simulink library "SUB_PLANT_Engine"  (R2018a)
settings: Solver=VariableStepAuto  StartTime=0.0  StopTime=10.0  RelTol=1e-3
libraries: PTC_MBDS_LIB x19, simulink x9
settings Model: Creator=Sundeep.Tuteja  LastModifiedBy=John.Lahti

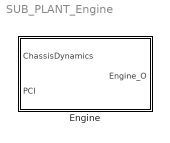
== system SUB_PLANT_Engine ==
  Engine : Subsystem

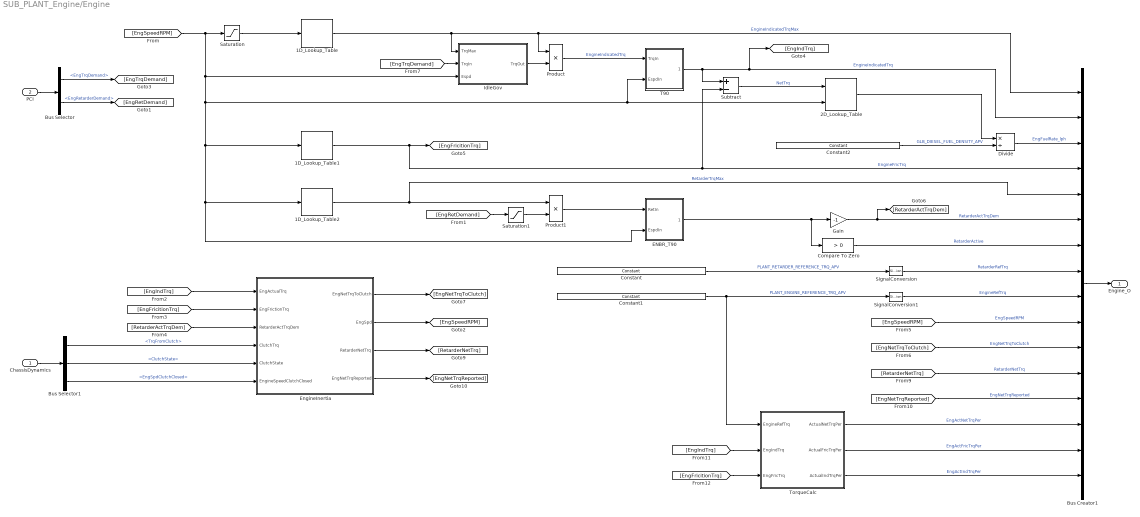
== system SUB_PLANT_Engine/Engine ==
  ChassisDynamics : Inport
  PCI : Inport  Port=2
  1D_Lookup_Table : PTC_MBDS_LIB/Extras/Lookup Tables/1D_Lookup_Table  ParameterObjectName=PLANT_ENGINE_INDICATED_TORQUE_DATA_MPV  InterpolationMethod=Linear  PTC_MBDS_BlockVersion=5.41  PTC_BlockType=PTC_MBDS_1D_Lookup_Table
      settings: SourceProductName=PACCAR Technical Center MBDS Library
      settings: AttributesFormatString=|
      | X Axis: PLANT_ENGINE_INDICATED_TORQUE_STEP_MPV (rpm)
      | Y Axis: PLANT_ENGINE_INDICATED_TORQUE_DATA_MPV (N*m)
      | Interpolation Method: Linear
  1D_Lookup_Table1 : PTC_MBDS_LIB/Extras/Lookup Tables/1D_Lookup_Table  ParameterObjectName=PLANT_ENGINE_FRICTION_TORQUE_DATA_MPV  InterpolationMethod=Linear  PTC_MBDS_BlockVersion=5.41  PTC_BlockType=PTC_MBDS_1D_Lookup_Table
      settings: SourceProductName=PACCAR Technical Center MBDS Library
      settings: AttributesFormatString=|
      | X Axis: PLANT_ENGINE_FRICTION_TORQUE_STEP_MPV (rpm)
      | Y Axis: PLANT_ENGINE_FRICTION_TORQUE_DATA_MPV (N*m)
      | Interpolation Method: Linear
  1D_Lookup_Table2 : PTC_MBDS_LIB/Extras/Lookup Tables/1D_Lookup_Table  ParameterObjectName=PLANT_RETARDER_TORQUE_DATA_MPV  InterpolationMethod=Linear  PTC_MBDS_BlockVersion=5.41  PTC_BlockType=PTC_MBDS_1D_Lookup_Table
      settings: SourceProductName=PACCAR Technical Center MBDS Library
      settings: AttributesFormatString=|
      | X Axis: PLANT_RETARDER_TORQUE_STEP_MPV (rpm)
      | Y Axis: PLANT_RETARDER_TORQUE_DATA_MPV (N*m)
      | Interpolation Method: Linear
  2D_Lookup_Table : PTC_MBDS_LIB/Extras/Lookup Tables/2D_Lookup_Table  ParameterObjectName=PLANT_ENGINE_FUEL_MAP_DATA_MPV  InterpolationMethod=Linear  PTC_MBDS_BlockVersion=5.41  PTC_BlockType=PTC_MBDS_2D_Lookup_Table
      settings: SourceProductName=PACCAR Technical Center MBDS Library
      settings: AttributesFormatString=|
      | Row Axis: PLANT_ENGINE_FUEL_MAP_TRQ_STEP_MPV (N*m)
      | Column Axis: PLANT_ENGINE_FUEL_MAP_ESPD_STEP_MPV (rpm)
      | Data Axis: PLANT_ENGINE_FUEL_MAP_DATA_MPV (kg/h)
      | Interpolation Method: Linear
  Bus Creator1 : BusCreator  Inputs=16
  Bus Selector : BusSelector  OutputSignals=EngTrqDemand,EngRetarderDemand
  Bus Selector1 : BusSelector  OutputSignals=Chassis.TrqFromClutch,Chassis.ClutchState,Chassis.EngSpdClutchClosed
  Compare To Zero : simulink/Logic and Bit Operations/Compare To Zero  relop=>  OutDataTypeStr=boolean
  Constant : PTC_MBDS_LIB/Extras/Sources/Constant  Value2=PLANT_RETARDER_REFERENCE_TRQ_APV  PTC_MBDS_BlockVersion=5.41  PTC_BlockType=PTC_MBDS_Constant
      settings: SourceProductName=PACCAR Technical Center MBDS Library
      settings: AttributesFormatString=|
      | Value: 1779
      | Unit: 'N*m'
  Constant1 : PTC_MBDS_LIB/Extras/Sources/Constant  Value2=PLANT_ENGINE_REFERENCE_TRQ_APV  PTC_MBDS_BlockVersion=5.41  PTC_BlockType=PTC_MBDS_Constant
      settings: SourceProductName=PACCAR Technical Center MBDS Library
      settings: AttributesFormatString=|
      | Value: 2374
      | Unit: 'N*m'
  Constant2 : PTC_MBDS_LIB/Extras/Sources/Constant  Value2=GLB_DIESEL_FUEL_DENSITY_APV  PTC_MBDS_BlockVersion=5.41  PTC_BlockType=PTC_MBDS_Constant
      settings: SourceProductName=PACCAR Technical Center MBDS Library
      settings: AttributesFormatString=|
      | Value: 0.8477
      | Unit: 'kg/L'
  Divide : Product  Inputs=*/  OutDataTypeStr=Inherit: Inherit via back propagation  SaturateOnIntegerOverflow=on  InputSameDT=on
      settings: AttributesFormatString=Saturate: %<SaturateOnIntegerOverflow>
  ENBR_T90 : Subsystem
  EngineInertia : Subsystem
  Gain : Gain  Gain=-1
  IdleGov : Subsystem
  Product : Product
  Product1 : Product
  Saturation : Saturate  UpperLimit=5000  LowerLimit=500
  Saturation1 : Saturate  UpperLimit=1  LowerLimit=0
  SignalConversion : SignalConversion  ConversionOutput=Contiguous copy  OverrideOpt=off
  SignalConversion1 : SignalConversion  ConversionOutput=Contiguous copy  OverrideOpt=off
  Subtract : Sum  Inputs=+-
  T90 : Subsystem
  TorqueCalc : Subsystem
  Engine_O : Outport
  wires:
  EngineInertia/4(EngNetTrqReported) -> [EngNetTrqReported]
  EngineInertia/3(RetarderNetTrq) -> [RetarderNetTrq]
  EngineInertia/2(EngSpd) -> [EngSpeedRPM]
  EngineInertia/1(EngNetTrqToClutch) -> [EngNetTrqToClutch]
  TorqueCalc/3(ActualIndTrqPer) -> Bus Creator1/16  "EngActIndTrqPer"
  SignalConversion1/1 -> Bus Creator1/9  "EngineRefTrq"
  SignalConversion/1 -> Bus Creator1/8  "RetarderRefTrq"
  TorqueCalc/2(ActualFricTrqPer) -> Bus Creator1/15  "EngActFricTrqPer"
  TorqueCalc/1(ActualNetTrqPer) -> Bus Creator1/14  "EngActNetTrqPer"
  [EngFricitionTrq] -> TorqueCalc/3(EngFricTrq)
  [EngIndTrq] -> TorqueCalc/2(EngIndTrq)
  [EngNetTrqReported] -> Bus Creator1/13  "EngNetTrqReported"
  [RetarderNetTrq] -> Bus Creator1/12  "RetarderNetTrq"
  [EngNetTrqToClutch] -> Bus Creator1/11  "EngNetTrqToClutch"
  [EngSpeedRPM] -> Bus Creator1/10  "EngSpeedRPM"
  Bus Selector1/3 -> EngineInertia/6(EngineSpeedClutchClosed)  "<EngSpdClutchClosed>"
  Bus Selector1/2 -> EngineInertia/5(ClutchState)  "<ClutchState>"
  Bus Selector1/1 -> EngineInertia/4(ClutchTrq)  "<TrqFromClutch>"
  ChassisDynamics/1 -> Bus Selector1/1
  [RetarderActTrqDem] -> EngineInertia/3(RetarderActTrqDem)
  [EngFricitionTrq] -> EngineInertia/2(EngFrictionTrq)
  [EngIndTrq] -> EngineInertia/1(EngActualTrq)
  1D_Lookup_Table1/1 -> Bus Creator1/4, Subtract/2, [EngFricitionTrq]  "EngineFricTrq"
  Bus Creator1/1 -> Engine_O/1
  Saturation/1 -> 1D_Lookup_Table/1
  1D_Lookup_Table/1 -> Bus Creator1/1, Product/1, IdleGov/1(TrqMax)  "EngineIndicatedTrqMax"
  1D_Lookup_Table2/1 -> Product1/1, Bus Creator1/5  "RetarderTrqMax"
  [EngRetDemand] -> Saturation1/1
  Saturation1/1 -> Product1/2
  Compare To Zero/1 -> Bus Creator1/7  "RetarderActive"
  Gain/1 -> Bus Creator1/6, [RetarderActTrqDem]  "RetarderActTrqDem"
  2D_Lookup_Table/1 -> Divide/1
  PCI/1 -> Bus Selector/1
  Bus Selector/1 -> [EngTrqDemand]  "<EngTrqDemand>"
  Bus Selector/2 -> [EngRetDemand]  "<EngRetarderDemand>"
  Subtract/1 -> 2D_Lookup_Table/1  "NetTrq"
  T90/1(TrqOut) -> [EngIndTrq], Bus Creator1/2, Subtract/1  "EngineIndicatedTrq"
  ENBR_T90/1(RetOut) -> Gain/1, Compare To Zero/1
  [EngSpeedRPM] -> Saturation/1, IdleGov/3(Espd), 2D_Lookup_Table/2, T90/2(EspdIn), 1D_Lookup_Table1/1, 1D_Lookup_Table2/1, ENBR_T90/2(EspdIn)
  Product/1 -> T90/1(TrqIn)  "EngineIndicatedTrq"
  Product1/1 -> ENBR_T90/1(RetIn)
  Divide/1 -> Bus Creator1/3  "EngFuelRate_lph"
  [EngTrqDemand] -> IdleGov/2(TrqIn)
  IdleGov/1(TrqOut) -> Product/2
  Constant/1 -> SignalConversion/1  "PLANT_RETARDER_REFERENCE_TRQ_APV"
  Constant1/1 -> TorqueCalc/1(EngineRefTrq), SignalConversion1/1  "PLANT_ENGINE_REFERENCE_TRQ_APV"
  Constant2/1 -> Divide/2  "GLB_DIESEL_FUEL_DENSITY_APV"

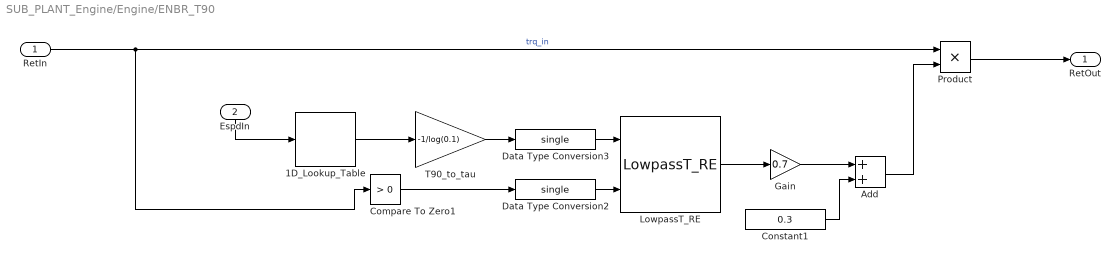
== system SUB_PLANT_Engine/Engine/ENBR_T90 ==
  RetIn : Inport
  EspdIn : Inport  Port=2
  1D_Lookup_Table : PTC_MBDS_LIB/Extras/Lookup Tables/1D_Lookup_Table  ParameterObjectName=PLANT_ENGINE_REV_T90_TIMES_MPV  InterpolationMethod=Linear  PTC_MBDS_BlockVersion=5.41  PTC_BlockType=PTC_MBDS_1D_Lookup_Table
      settings: SourceProductName=PACCAR Technical Center MBDS Library
      settings: AttributesFormatString=|
      | X Axis: PLANT_ENGINE_REV_T90_TIMES_ESPD_STEP_MPV (rpm)
      | Y Axis: PLANT_ENGINE_REV_T90_TIMES_MPV (s)
      | Interpolation Method: Linear
  Add : Sum
  Compare To Zero1 : simulink/Logic and Bit Operations/Compare To Zero  relop=>  OutDataTypeStr=boolean
  Constant1 : Constant  Value=0.3  OutDataTypeStr=single
  Data Type Conversion2 : DataTypeConversion  OutDataTypeStr=single
  Data Type Conversion3 : DataTypeConversion  OutDataTypeStr=single
  Gain : Gain  Gain=0.7
  LowpassT_RE : PTC_MBDS_LIB/MBDS Standard Library/Extended Operations/Filters/LowpassT_RE  dT_Enabled=off  dT=GLB_FIXED_STEP_SIZE_CPV  E_Enabled=off  R_Enabled=off  IV_Enabled=off  IV=0  PTC_MBDS_BlockVersion=5.41  PTC_BlockType=PTC_MBDS_LowpassT_RE
      settings: SourceProductName=PACCAR Technical Center MBDS Library
      settings: AttributesFormatString=|
      | IV = %<IV>
      | dT = %<dT>
  Product : Product
  T90_to_tau : Gain  Gain=-1/log(0.1)
  RetOut : Outport
  wires:
  Data Type Conversion2/1 -> LowpassT_RE/2
  Data Type Conversion3/1 -> LowpassT_RE/1
  1D_Lookup_Table/1 -> T90_to_tau/1
  EspdIn/1 -> 1D_Lookup_Table/1
  T90_to_tau/1 -> Data Type Conversion3/1
  Product/1 -> RetOut/1
  RetIn/1 -> Product/1, Compare To Zero1/1  "trq_in"
  Compare To Zero1/1 -> Data Type Conversion2/1
  Gain/1 -> Add/1
  Constant1/1 -> Add/2
  Add/1 -> Product/2
  LowpassT_RE/1 -> Gain/1

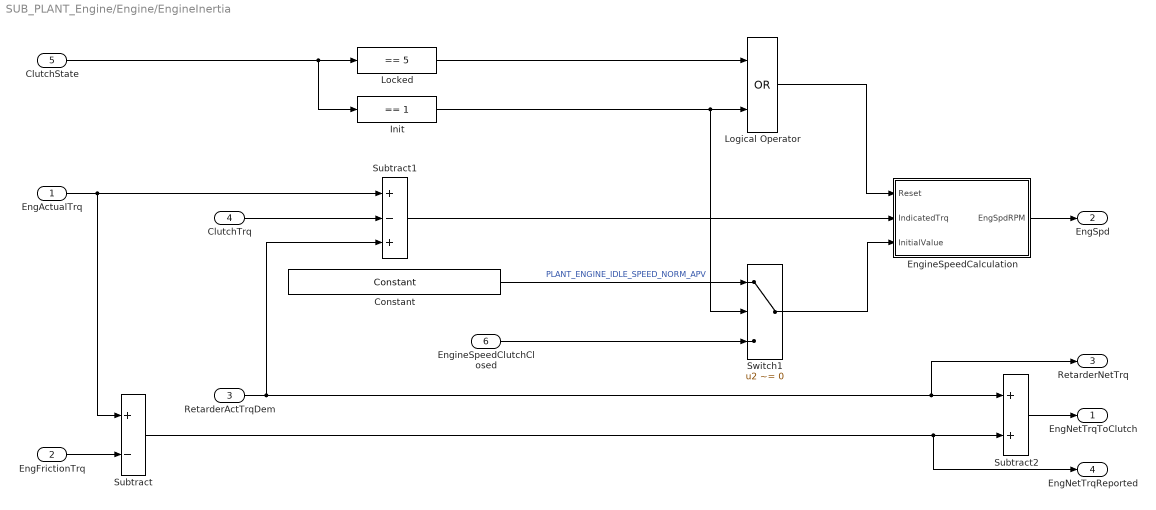
== system SUB_PLANT_Engine/Engine/EngineInertia ==
  EngActualTrq : Inport
  EngFrictionTrq : Inport  Port=2
  RetarderActTrqDem : Inport  Port=3
  ClutchTrq : Inport  Port=4
  ClutchState : Inport  Port=5
  EngineSpeedClutchClosed : Inport  Port=6
  Constant : PTC_MBDS_LIB/Extras/Sources/Constant  Value2=PLANT_ENGINE_IDLE_SPEED_NORM_APV  PTC_MBDS_BlockVersion=5.41  PTC_BlockType=PTC_MBDS_Constant
      settings: SourceProductName=PACCAR Technical Center MBDS Library
      settings: AttributesFormatString=|
      | Value: 650
      | Unit: 'rpm'
  EngineSpeedCalculation : Subsystem
  Init : simulink/Logic and Bit Operations/Compare To Constant  relop===  const=1  OutDataTypeStr=boolean
  Locked : simulink/Logic and Bit Operations/Compare To Constant  relop===  const=5  OutDataTypeStr=boolean
  Logical Operator : Logic  Operator=OR  AllPortsSameDT=off  OutDataTypeStr=boolean
  Subtract : Sum  Inputs=+-
  Subtract1 : Sum  Inputs=+-+
  Subtract2 : Sum
  Switch1 : Switch  Criteria=u2 ~= 0
  EngNetTrqToClutch : Outport
  EngSpd : Outport  Port=2
  RetarderNetTrq : Outport  Port=3
  EngNetTrqReported : Outport  Port=4
  wires:
  Constant/1 -> Switch1/1  "PLANT_ENGINE_IDLE_SPEED_NORM_APV"
  Subtract1/1 -> EngineSpeedCalculation/2(IndicatedTrq)
  RetarderActTrqDem/1 -> Subtract2/1, RetarderNetTrq/1, Subtract1/3
  Subtract2/1 -> EngNetTrqToClutch/1
  EngineSpeedCalculation/1(EngSpdRPM) -> EngSpd/1
  Logical Operator/1 -> EngineSpeedCalculation/1(Reset)
  Locked/1 -> Logical Operator/1
  ClutchState/1 -> Init/1, Locked/1
  ClutchTrq/1 -> Subtract1/2
  EngFrictionTrq/1 -> Subtract/2
  EngActualTrq/1 -> Subtract1/1, Subtract/1
  Subtract/1 -> Subtract2/2, EngNetTrqReported/1
  Init/1 -> Switch1/2, Logical Operator/2
  EngineSpeedClutchClosed/1 -> Switch1/3
  Switch1/1 -> EngineSpeedCalculation/3(InitialValue)

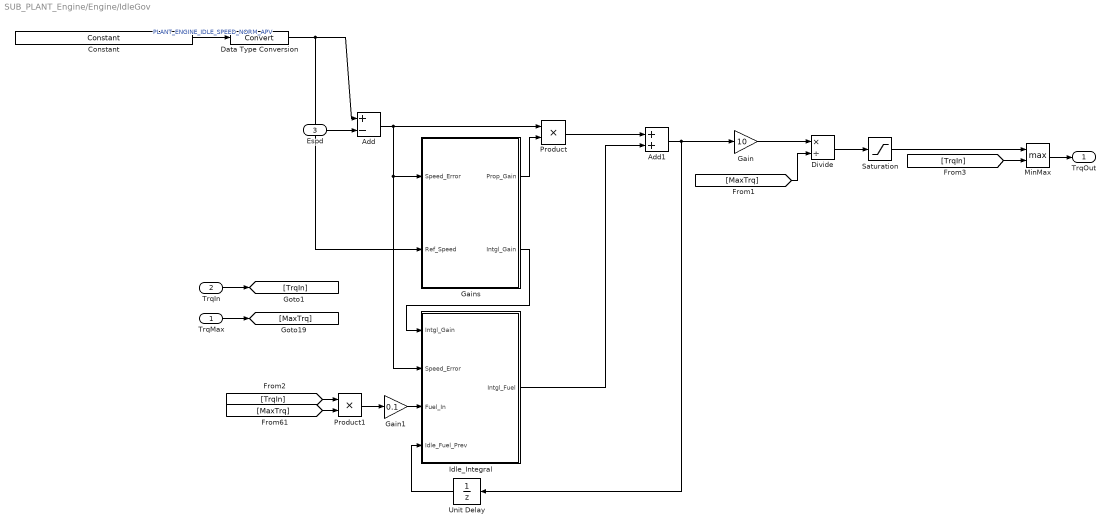
== system SUB_PLANT_Engine/Engine/IdleGov ==
  TrqMax : Inport
  TrqIn : Inport  Port=2
  Espd : Inport  Port=3
  Add : Sum  Inputs=+-
  Add1 : Sum
  Constant : PTC_MBDS_LIB/Extras/Sources/Constant  Value2=PLANT_ENGINE_IDLE_SPEED_NORM_APV  PTC_MBDS_BlockVersion=5.41  PTC_BlockType=PTC_MBDS_Constant
      settings: SourceProductName=PACCAR Technical Center MBDS Library
      settings: AttributesFormatString=|
      | Value: 650
      | Unit: 'rpm'
  Data Type Conversion : DataTypeConversion  SaturateOnIntegerOverflow=on
  Divide : Product  Inputs=*/
  Gain : Gain  Gain=10
  Gain1 : Gain  Gain=0.1
  Gains : Subsystem
  Idle_Integral : Subsystem
  MinMax : MinMax  Function=max  Inputs=2
  Product : Product
  Product1 : Product
  Saturation : Saturate  UpperLimit=1  LowerLimit=0
  Unit Delay : UnitDelay  SampleTime=-1
  TrqOut : Outport
  wires:
  Constant/1 -> Data Type Conversion/1  "PLANT_ENGINE_IDLE_SPEED_NORM_APV"
  Espd/1 -> Add/2
  Add/1 -> Product/1, Gains/1(Speed_Error), Idle_Integral/2(Speed_Error)
  Product/1 -> Add1/1
  Add1/1 -> Unit Delay/1, Gain/1
  Gain/1 -> Divide/1
  Divide/1 -> Saturation/1
  Gains/1(Prop_Gain) -> Product/2
  TrqMax/1 -> [MaxTrq]
  [MaxTrq] -> Divide/2
  [MaxTrq] -> Product1/2
  Product1/1 -> Gain1/1
  Gain1/1 -> Idle_Integral/3(Fuel_In)
  Gains/2(Intgl_Gain) -> Idle_Integral/1(Intgl_Gain)
  Idle_Integral/1(Intgl_Fuel) -> Add1/2
  TrqIn/1 -> [TrqIn]
  [TrqIn] -> Product1/1
  Unit Delay/1 -> Idle_Integral/4(Idle_Fuel_Prev)
  [TrqIn] -> MinMax/2
  Saturation/1 -> MinMax/1
  MinMax/1 -> TrqOut/1
  Data Type Conversion/1 -> Gains/2(Ref_Speed), Add/1

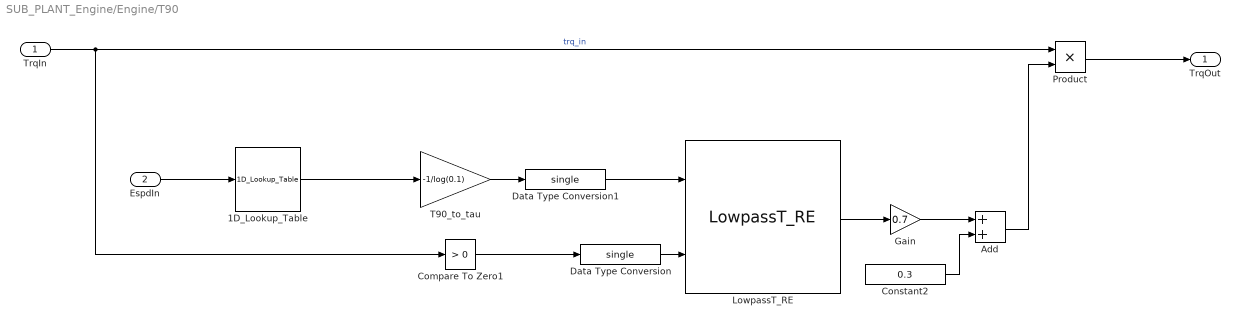
== system SUB_PLANT_Engine/Engine/T90 ==
  TrqIn : Inport  OutDataTypeStr=double
  EspdIn : Inport  Port=2
  1D_Lookup_Table : PTC_MBDS_LIB/Extras/Lookup Tables/1D_Lookup_Table  ParameterObjectName=PLANT_ENGINE_T90_TIMES_MPV  InterpolationMethod=Linear  PTC_MBDS_BlockVersion=5.41  PTC_BlockType=PTC_MBDS_1D_Lookup_Table
      settings: SourceProductName=PACCAR Technical Center MBDS Library
      settings: AttributesFormatString=|
      | X Axis: PLANT_ENGINE_T90_TIMES_ESPD_STEP_MPV (rpm)
      | Y Axis: PLANT_ENGINE_T90_TIMES_MPV (s)
      | Interpolation Method: Linear
  Add : Sum
  Compare To Zero1 : simulink/Logic and Bit Operations/Compare To Zero  relop=>  OutDataTypeStr=boolean
  Constant2 : Constant  Value=0.3  OutDataTypeStr=single
  Data Type Conversion : DataTypeConversion  OutDataTypeStr=single
  Data Type Conversion1 : DataTypeConversion  OutDataTypeStr=single
  Gain : Gain  Gain=0.7
  LowpassT_RE : PTC_MBDS_LIB/MBDS Standard Library/Extended Operations/Filters/LowpassT_RE  dT_Enabled=off  dT=GLB_FIXED_STEP_SIZE_CPV  E_Enabled=off  R_Enabled=off  IV_Enabled=off  IV=0  PTC_MBDS_BlockVersion=5.41  PTC_BlockType=PTC_MBDS_LowpassT_RE
      settings: SourceProductName=PACCAR Technical Center MBDS Library
      settings: AttributesFormatString=|
      | IV = %<IV>
      | dT = %<dT>
  Product : Product
  T90_to_tau : Gain  Gain=-1/log(0.1)
  TrqOut : Outport
  wires:
  Product/1 -> TrqOut/1
  Data Type Conversion/1 -> LowpassT_RE/2
  Data Type Conversion1/1 -> LowpassT_RE/1
  T90_to_tau/1 -> Data Type Conversion1/1
  EspdIn/1 -> 1D_Lookup_Table/1
  TrqIn/1 -> Compare To Zero1/1, Product/1  "trq_in"
  1D_Lookup_Table/1 -> T90_to_tau/1
  Compare To Zero1/1 -> Data Type Conversion/1
  LowpassT_RE/1 -> Gain/1
  Gain/1 -> Add/1
  Constant2/1 -> Add/2
  Add/1 -> Product/2

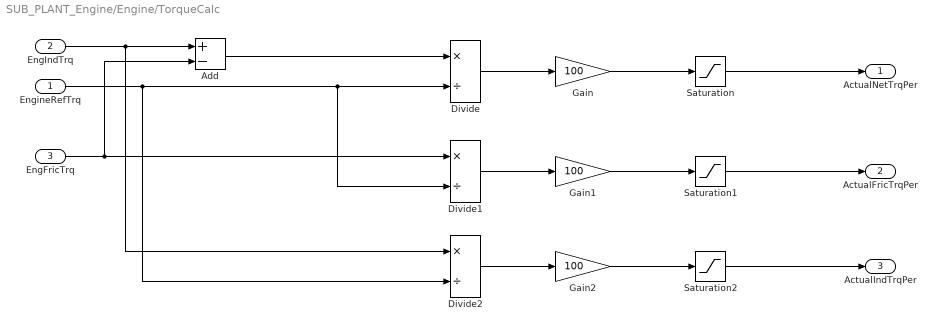
== system SUB_PLANT_Engine/Engine/TorqueCalc ==
  EngineRefTrq : Inport
  EngIndTrq : Inport  Port=2
  EngFricTrq : Inport  Port=3
  Add : Sum  Inputs=+-
  Divide : Product  Inputs=*/
  Divide1 : Product  Inputs=*/
  Divide2 : Product  Inputs=*/
  Gain : Gain  Gain=100
  Gain1 : Gain  Gain=100
  Gain2 : Gain  Gain=100
  Saturation : Saturate  UpperLimit=100  LowerLimit=-100
      settings: AttributesFormatString=|
      | Max = %<UpperLimit>
      | Min = %<LowerLimit>
  Saturation1 : Saturate  UpperLimit=100  LowerLimit=0
      settings: AttributesFormatString=|
      | Max = %<UpperLimit>
      | Min = %<LowerLimit>
  Saturation2 : Saturate  UpperLimit=100  LowerLimit=0
      settings: AttributesFormatString=|
      | Max = %<UpperLimit>
      | Min = %<LowerLimit>
  ActualNetTrqPer : Outport
  ActualFricTrqPer : Outport  Port=2
  ActualIndTrqPer : Outport  Port=3
  wires:
  Saturation2/1 -> ActualIndTrqPer/1
  Gain2/1 -> Saturation2/1
  Divide2/1 -> Gain2/1
  EngineRefTrq/1 -> Divide/2, Divide1/2, Divide2/2
  Saturation1/1 -> ActualFricTrqPer/1
  Gain1/1 -> Saturation1/1
  Divide1/1 -> Gain1/1
  Saturation/1 -> ActualNetTrqPer/1
  EngFricTrq/1 -> Divide1/1, Add/2
  EngIndTrq/1 -> Add/1, Divide2/1
  Gain/1 -> Saturation/1
  Divide/1 -> Gain/1
  Add/1 -> Divide/1

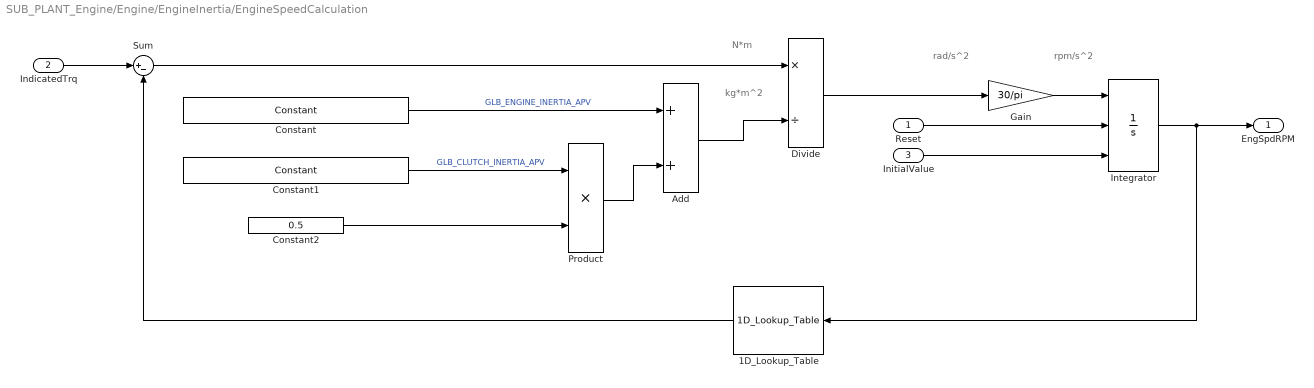
== system SUB_PLANT_Engine/Engine/EngineInertia/EngineSpeedCalculation ==
  note: kg*m^2
  note: N*m
  note: rpm/s^2
  note: rad/s^2
  Reset : Inport
  IndicatedTrq : Inport  Port=2
  InitialValue : Inport  Port=3
  1D_Lookup_Table : PTC_MBDS_LIB/Extras/Lookup Tables/1D_Lookup_Table  ParameterObjectName=PLANT_ENGINE_FRICTION_TORQUE_DATA_MPV  InterpolationMethod=Linear  PTC_MBDS_BlockVersion=5.41  PTC_BlockType=PTC_MBDS_1D_Lookup_Table
      settings: SourceProductName=PACCAR Technical Center MBDS Library
      settings: AttributesFormatString=|
      | X Axis: PLANT_ENGINE_FRICTION_TORQUE_STEP_MPV (rpm)
      | Y Axis: PLANT_ENGINE_FRICTION_TORQUE_DATA_MPV (N*m)
      | Interpolation Method: Linear
  Add : Sum  OutDataTypeStr=Inherit: Inherit via back propagation  SaturateOnIntegerOverflow=on  InputSameDT=on
      settings: AttributesFormatString=Saturate: %<SaturateOnIntegerOverflow>
  Constant : PTC_MBDS_LIB/Extras/Sources/Constant  Value2=GLB_ENGINE_INERTIA_APV  PTC_MBDS_BlockVersion=5.41  PTC_BlockType=PTC_MBDS_Constant
      settings: SourceProductName=PACCAR Technical Center MBDS Library
      settings: AttributesFormatString=|
      | Value: 3.7109375
      | Unit: 'kg*m^2'
  Constant1 : PTC_MBDS_LIB/Extras/Sources/Constant  Value2=GLB_CLUTCH_INERTIA_APV  PTC_MBDS_BlockVersion=5.41  PTC_BlockType=PTC_MBDS_Constant
      settings: SourceProductName=PACCAR Technical Center MBDS Library
      settings: AttributesFormatString=|
      | Value: 0.115966796875
      | Unit: 'kg*m^2'
  Constant2 : Constant  Value=0.5
  Divide : Product  Inputs=*/  OutDataTypeStr=Inherit: Inherit via back propagation  SaturateOnIntegerOverflow=on  InputSameDT=on
      settings: AttributesFormatString=Saturate: %<SaturateOnIntegerOverflow>
  Gain : Gain  Gain=30/pi
  Integrator : Integrator  ExternalReset=level  InitialConditionSource=external  InitialCondition=650  LimitOutput=on  UpperSaturationLimit=10000  LowerSaturationLimit=0
  Product : Product  Inputs=**  OutDataTypeStr=Inherit: Inherit via back propagation  SaturateOnIntegerOverflow=on  InputSameDT=on
      settings: AttributesFormatString=Saturate: %<SaturateOnIntegerOverflow>
  Sum : Sum  Inputs=|+-
  EngSpdRPM : Outport
  wires:
  Constant2/1 -> Product/2
  Constant1/1 -> Product/1  "GLB_CLUTCH_INERTIA_APV"
  Constant/1 -> Add/1  "GLB_ENGINE_INERTIA_APV"
  InitialValue/1 -> Integrator/3
  IndicatedTrq/1 -> Sum/1
  1D_Lookup_Table/1 -> Sum/2
  Sum/1 -> Divide/1
  Divide/1 -> Gain/1
  Reset/1 -> Integrator/2
  Integrator/1 -> EngSpdRPM/1, 1D_Lookup_Table/1
  Gain/1 -> Integrator/1
  Product/1 -> Add/2
  Add/1 -> Divide/2

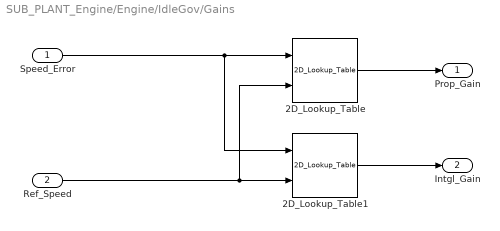
== system SUB_PLANT_Engine/Engine/IdleGov/Gains ==
  Speed_Error : Inport
  Ref_Speed : Inport  Port=2
  2D_Lookup_Table : PTC_MBDS_LIB/Extras/Lookup Tables/2D_Lookup_Table  ParameterObjectName=PLANT_ENGINE_IDLE_GOV_GAINS_PROP_MPV  InterpolationMethod=Linear  PTC_MBDS_BlockVersion=5.41  PTC_BlockType=PTC_MBDS_2D_Lookup_Table
      settings: SourceProductName=PACCAR Technical Center MBDS Library
      settings: AttributesFormatString=|
      | Row Axis: PLANT_ENGINE_IDLE_GOV_GAINS_Y_MPV (km/h)
      | Column Axis: PLANT_ENGINE_IDLE_GOV_GAINS_X_MPV (rpm)
      | Data Axis: PLANT_ENGINE_IDLE_GOV_GAINS_PROP_MPV (1)
      | Interpolation Method: Linear
  2D_Lookup_Table1 : PTC_MBDS_LIB/Extras/Lookup Tables/2D_Lookup_Table  ParameterObjectName=PLANT_ENGINE_IDLE_GOV_GAINS_INTGL_MPV  InterpolationMethod=Linear  PTC_MBDS_BlockVersion=5.41  PTC_BlockType=PTC_MBDS_2D_Lookup_Table
      settings: SourceProductName=PACCAR Technical Center MBDS Library
      settings: AttributesFormatString=|
      | Row Axis: PLANT_ENGINE_IDLE_GOV_GAINS_Y_MPV (km/h)
      | Column Axis: PLANT_ENGINE_IDLE_GOV_GAINS_X_MPV (rpm)
      | Data Axis: PLANT_ENGINE_IDLE_GOV_GAINS_INTGL_MPV (1/s)
      | Interpolation Method: Linear
  Prop_Gain : Outport
  Intgl_Gain : Outport  Port=2
  wires:
  2D_Lookup_Table/1 -> Prop_Gain/1
  2D_Lookup_Table1/1 -> Intgl_Gain/1
  Speed_Error/1 -> 2D_Lookup_Table1/1, 2D_Lookup_Table/1
  Ref_Speed/1 -> 2D_Lookup_Table1/2, 2D_Lookup_Table/2

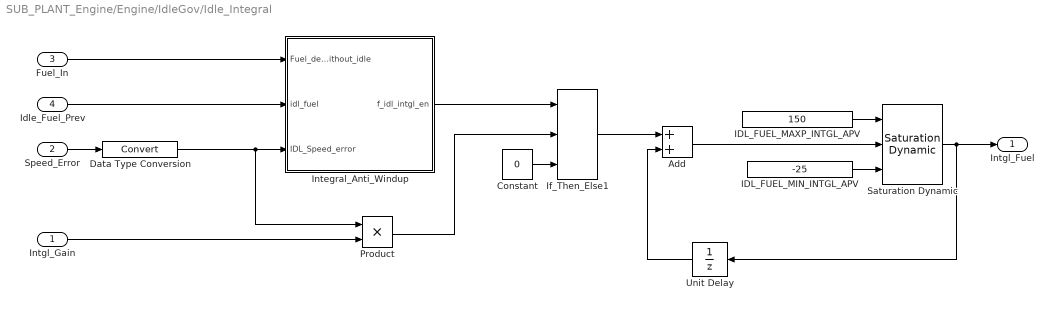
== system SUB_PLANT_Engine/Engine/IdleGov/Idle_Integral ==
  Intgl_Gain : Inport
  Speed_Error : Inport  Port=2
  Fuel_In : Inport  Port=3
  Idle_Fuel_Prev : Inport  Port=4
  Add : Sum
  Constant : Constant  Value=0
  Data Type Conversion : DataTypeConversion  SaturateOnIntegerOverflow=on
  IDL_FUEL_MAXP_INTGL_APV : Constant  Value=150
  IDL_FUEL_MIN_INTGL_APV : Constant  Value=-25
  If_Then_Else1 : PTC_MBDS_LIB/Extras/Signal Routing/If_Then_Else  PTC_MBDS_BlockVersion=5.41  PTC_BlockType=PTC_MBDS_If_Then_Else
      settings: SourceProductName=PACCAR Technical Center MBDS Library
  Integral_Anti_Windup : Subsystem
  Product : Product
  Saturation Dynamic : simulink/Discontinuities/Saturation Dynamic  OutMin=[]  OutMax=[]  OutDataTypeStr=Inherit: Same as second input  OutDataType=fixdt(1, 16)  OutScaling=2^-10  DoSatur=off
  Unit Delay : UnitDelay  InitialCondition=40  SampleTime=-1
  Intgl_Fuel : Outport
  wires:
  Fuel_In/1 -> Integral_Anti_Windup/1(Fuel_demand_without_idle)
  Speed_Error/1 -> Data Type Conversion/1
  Idle_Fuel_Prev/1 -> Integral_Anti_Windup/2(idl_fuel)
  Intgl_Gain/1 -> Product/2
  Integral_Anti_Windup/1(f_idl_intgl_en) -> If_Then_Else1/1
  Product/1 -> If_Then_Else1/2
  Constant/1 -> If_Then_Else1/3
  If_Then_Else1/1 -> Add/1
  Unit Delay/1 -> Add/2
  Add/1 -> Saturation Dynamic/2
  Saturation Dynamic/1 -> Unit Delay/1, Intgl_Fuel/1
  IDL_FUEL_MAXP_INTGL_APV/1 -> Saturation Dynamic/1
  IDL_FUEL_MIN_INTGL_APV/1 -> Saturation Dynamic/3
  Data Type Conversion/1 -> Product/1, Integral_Anti_Windup/3(IDL_Speed_error)

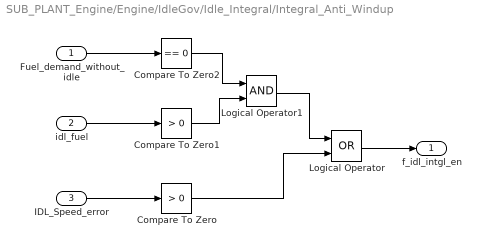
== system SUB_PLANT_Engine/Engine/IdleGov/Idle_Integral/Integral_Anti_Windup ==
  Fuel_demand_without_idle : Inport
  idl_fuel : Inport  Port=2
  IDL_Speed_error : Inport  Port=3
  Compare To Zero : simulink/Logic and Bit Operations/Compare To Zero  relop=>  OutDataTypeStr=boolean
  Compare To Zero1 : simulink/Logic and Bit Operations/Compare To Zero  relop=>  OutDataTypeStr=boolean
  Compare To Zero2 : simulink/Logic and Bit Operations/Compare To Zero  relop===  OutDataTypeStr=boolean
  Logical Operator : Logic  Operator=OR  AllPortsSameDT=off  OutDataTypeStr=boolean
  Logical Operator1 : Logic  AllPortsSameDT=off  OutDataTypeStr=boolean
  f_idl_intgl_en : Outport
  wires:
  Logical Operator/1 -> f_idl_intgl_en/1
  IDL_Speed_error/1 -> Compare To Zero/1
  Compare To Zero/1 -> Logical Operator/2
  Logical Operator1/1 -> Logical Operator/1
  Compare To Zero1/1 -> Logical Operator1/2
  Compare To Zero2/1 -> Logical Operator1/1
  Fuel_demand_without_idle/1 -> Compare To Zero2/1
  idl_fuel/1 -> Compare To Zero1/1
